simulink model "RequirementsTable1"  (R2023a)
settings: Solver=VariableStepAuto  StartTime=0.0  StopTime=10.0  RelTol=1e-3
settings Model: Creator=bened  LastModifiedBy=bened

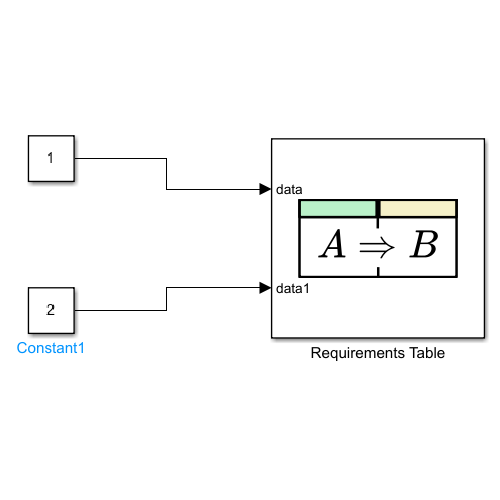
[thumbnail: Simulink's stored preview of the top-level diagram]
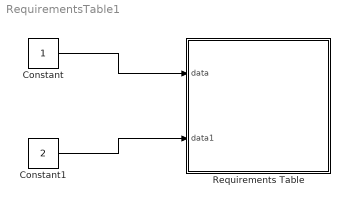
== system RequirementsTable1 ==
  Constant : Constant
  Constant1 : Constant  Value=2
  Requirements Table : Requirements Table  TreatAsAtomicUnit=on
  wires:
  Constant/1 -> Requirements Table/1(data)
  Constant1/1 -> Requirements Table/2(data1)

== stateflow chart RequirementsTable1/Requirements Table ==
  (default) -> (junction 1073741860)
  (junction 1073741860) -> (junction 1073741861) : {
      | % SF_REQ_REV_07
      | }
  (junction 1073741861) -> (junction 1073741863) : {
      | % HEADER_ASSIGNMENTS
      |
      | }
  (junction 1073741863) -> (junction 1073741865) : {
      | % START_A_4
      | }
  (junction 1073741865) -> (junction 1073741867) : {
      | }
  (junction 1073741867) -> (junction 1073741869)
  (junction 1073741869) -> (junction 1073741871) : {
      | }
  (junction 1073741871) -> (junction 1073741873) : {
      | % END_A_4
      | }
  (junction 1073741873) -> (junction 1073741910) : {
      | % START_R_1
      | }
  (junction 1073741910) -> (junction 1073741912) : {
      | }
  (junction 1073741912) -> (junction 1073741914)
  (junction 1073741914) -> (junction 1073741916) [order 1] : [(data>0)]
  (junction 1073741914) -> (junction 1073741922) [order 2]
  (junction 1073741916) -> (junction 1073741918) : {
      | y1=2*data
      |
      | }
  (junction 1073741918) -> (junction 1073741920) : {
      | }
  (junction 1073741920) -> (junction 1073741922)
  (junction 1073741922) -> (junction 1073741924)
  (junction 1073741924) -> (junction 1073741926) : {
      | % END_R_1
      | }
  (junction 1073741926) -> (junction 1073741943) : {
      | % START_R_7
      | }
  (junction 1073741943) -> (junction 1073741945) : {
      | }
  (junction 1073741945) -> (junction 1073741947)
  (junction 1073741947) -> (junction 1073741949) [order 1] : [(data1)]
  (junction 1073741947) -> (junction 1073741955) [order 2]
  (junction 1073741949) -> (junction 1073741951) : {
      | y2=0.5*data1
      |
      | }
  (junction 1073741951) -> (junction 1073741953) : {
      | }
  (junction 1073741953) -> (junction 1073741955)
  (junction 1073741955) -> (junction 1073741957)
  (junction 1073741957) -> (junction 1073741959) : {
      | % END_R_7
      | }
  data: data input; data1 input
